simulink model "exercitiul1colocviuTS2"  (R2021b)
settings: Solver=VariableStepAuto  StartTime=0.0  StopTime=10.0  RelTol=1e-3
undefined symbols (not defined in the file or in its folder): A, B, C

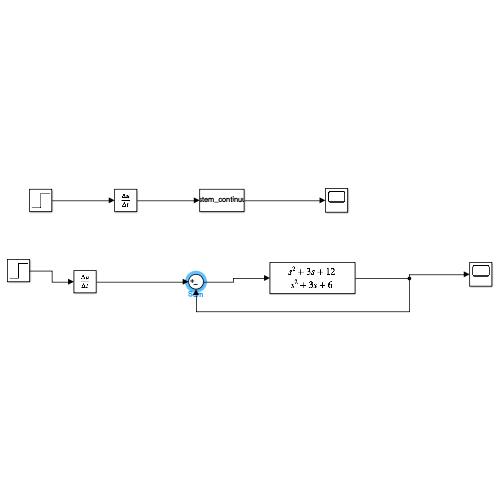
[thumbnail: Simulink's stored preview of the top-level diagram]
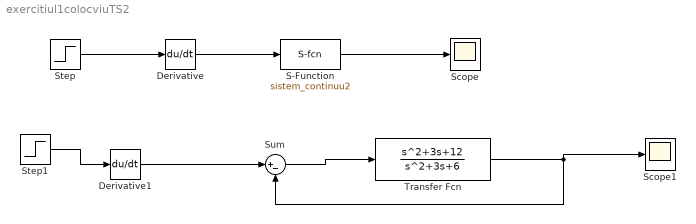
== system exercitiul1colocviuTS2 ==
  Derivative : Derivative
  Derivative1 : Derivative
  S-Function : S-Function  FunctionName=sistem_continuu2  Parameters=A,B,C  SFunctionDeploymentMode=off  EnableBusSupport=off
  Scope : Scope
  Scope1 : Scope
  Step : Step  SampleTime=0
  Step1 : Step  SampleTime=0
  Sum : Sum  Inputs=|+-
  Transfer Fcn : TransferFcn  Numerator=[1,3,12]  Denominator=[1 3 6]
  wires:
  Derivative/1 -> S-Function/1
  S-Function/1 -> Scope/1
  Sum/1 -> Transfer Fcn/1
  Transfer Fcn/1 -> Sum/2, Scope1/1
  Step/1 -> Derivative/1
  Derivative1/1 -> Sum/1
  Step1/1 -> Derivative1/1
